simulink model "playback_data"  (R2015a)
settings: Solver=FixedStepDiscrete  SolverMode=SingleTasking  StartTime=44  StopTime=72  FixedStep=sample_time  RelTol=1e-3
undefined symbols (not defined in the file or in its folder): A_kalman_no_position, A_kalman_transverse, A_kalman_vertical, A_lpf_10hz_05d, A_lpf_accelerometer, A_lpf_fourbar_angles, A_lpf_imu, A_lpf_lateral_angle, B1_lpf_10hz_05d, B1_lpf_accelerometer, B1_lpf_fourbar_angles, B1_lpf_imu, B1_lpf_lateral_angle, B2_lpf_10hz_05d, B2_lpf_accelerometer, B2_lpf_fourbar_angles, B2_lpf_imu, B2_lpf_lateral_angle, B_dx_versus_x0, B_kalman_no_position, B_kalman_transverse, B_kalman_vertical, backwards_K_sag_of_t, backwards_P_sag_of_t, boom_mount_angle, C_kalman_no_position, C_kalman_transverse, C_kalman_vertical, com_leg_motor, com_torso, contact_threshold, control_start_time, d_ankle_to_foot, d_vertical_boom_com_offset, d_vertical_com, desired_com_forward_velocity, desired_com_lateral_velocity, desired_initial_leg_roll_left, desired_initial_leg_roll_right, desired_standing_torso_pitch, desired_standing_torso_roll, desired_standing_z, desired_torso_pitch, desired_torso_roll, Discrete, enable_bouncing, fcut_contact, fdesignblkfcn, forward_dx_of_dxstar, forward_x_of_dxstar, g, gcbh, h_boom, HIP_MTR_MAX_CONT_TORQUE, HIP_MTR_MAX_TORQUE, i_leg_motor, i_robot, i_torso, initial_dx_estimate, initial_dx_takeoff_history ... (+82)
libraries: simulink x23, ctrlSharedLib x4, dsparch4 x3, dspfdesign x1
(part 2 of 6)

== system playback_data/Control/Behavior Control/Atrias Swing control ==
  note: Convert to
      | four-bar angles
  note: Position control the
      | individual four bar segments
  X Desired [m m/s m/s^2] : Inport
  Y Desired [m m/s m/s^2] : Inport  Port=2
  Z Desired [m m/s m/s^2] : Inport  Port=3
  Secondary Front Gear [rad rad/s] : Inport  Port=4
  Secondary Back Gear [rad rad/s] : Inport  Port=5
  Right or Left Stance [1 or 0] : Inport  Port=6
  Secondary Leg Roll [rad rad/s] : Inport  Port=7
  Secondary Leg Length [m m/s] : Inport  Port=8
  Secondary Leg Angle [rad rad/s] : Inport  Port=9
  Torso Pitch [rad rad/s] : Inport  Port=10
  Torso Roll [rad rad/s] : Inport  Port=11
  Pelvis to COM Position [m m m] : Inport  Port=12
  Pelvis to COM Velocity [m/s m/s m/s] : Inport  Port=13
  Avoid Hitting Mechanical Limits : MATLAB Function  TreatAsAtomicUnit=on
  Back / Front Velocity Tracking : Scope  NumInputPorts=2
      settings: YMin=-0.75~-5  YMax=3.25~1.5  SaveName=ScopeData36  SampleInput=on
  Back/Front PD : Subsystem
  "Convert COM Position to Joint Angles + Leg Length " : MATLAB Function  TreatAsAtomicUnit=on
  Demux4 : Demux  Outputs=2
  Demux5 : Demux  Outputs=2
  Demux6 : Demux  Outputs=6
  Mux{3..6,8,11..13} (8 alike) : Mux  Inputs=2
  Selector1 : Selector  InputPortWidth=2  Indices=[1]
  Selector2 : Selector  InputPortWidth=2  Indices=[1]
  Selector7 : Selector  InputPortWidth=2  Indices=[2]
  Selector8 : Selector  InputPortWidth=2  Indices=[2]
  Terminator : Terminator
  Two Pole Filter : DiscreteTransferFcn  Numerator=[A_lpf_10hz_05d 0 0]  Denominator=[1 B1_lpf_10hz_05d B2_lpf_10hz_05d]  SampleTime=sample_time
  Virtual Leg to Four Bar : MATLAB Function  TreatAsAtomicUnit=on
  Secondary Back/Front Motor Velocity [rad/s rad/s] : Outport
  Desired Swing Beta [rad rad/s rad/s^2] : Outport  Port=2
  wires:
  Two Pole Filter/1 -> Secondary Back/Front Motor Velocity [rad/s rad/s]/1
  Selector8/1 -> Mux12/2
  Selector7/1 -> Mux12/1
  Selector2/1 -> Mux13/2
  Selector1/1 -> Mux13/1
  Mux13/1 -> Back / Front Velocity Tracking/1
  Mux12/1 -> Back / Front Velocity Tracking/2
  Back/Front PD/1(Commanded Velocity [rad/s] [back front]) -> Selector2/1, Selector8/1, Two Pole Filter/1
  "Convert COM Position to Joint Angles + Leg Length "/3(desired_beta) -> Desired Swing Beta [rad rad/s rad/s^2]/1
  Pelvis to COM Velocity [m/s m/s m/s]/1 -> "Convert COM Position to Joint Angles + Leg Length "/6(dcom_pelvis_body)
  Pelvis to COM Position [m m m]/1 -> "Convert COM Position to Joint Angles + Leg Length "/5(com_pelvis_body)
  Mux5/1 -> Terminator/1
  Virtual Leg to Four Bar/5(dfront) -> Avoid Hitting Mechanical Limits/5(dfront_desired)
  Y Desired [m m/s m/s^2]/1 -> "Convert COM Position to Joint Angles + Leg Length "/2(Y_star)
  Mux8/1 -> Demux6/1
  "Convert COM Position to Joint Angles + Leg Length "/1(desired_leg_length) -> Mux8/1
  X Desired [m m/s m/s^2]/1 -> "Convert COM Position to Joint Angles + Leg Length "/1(X_star)
  Secondary Leg Length [m m/s]/1 -> "Convert COM Position to Joint Angles + Leg Length "/11(leg_length)
  "Convert COM Position to Joint Angles + Leg Length "/2(desired_alpha) -> Mux8/2
  Secondary Leg Angle [rad rad/s]/1 -> "Convert COM Position to Joint Angles + Leg Length "/9(sagittal_angle)
  Secondary Leg Roll [rad rad/s]/1 -> "Convert COM Position to Joint Angles + Leg Length "/10(lateral_angle)  "swing hip angle (lateral)"
  Right or Left Stance [1 or 0]/1 -> "Convert COM Position to Joint Angles + Leg Length "/4(right_left)
  Torso Roll [rad rad/s]/1 -> "Convert COM Position to Joint Angles + Leg Length "/7(roll)
  Torso Pitch [rad rad/s]/1 -> "Convert COM Position to Joint Angles + Leg Length "/8(pitch)
  Virtual Leg to Four Bar/1(back) -> Avoid Hitting Mechanical Limits/1(back_desired)
  Demux4/2 -> Mux11/2
  Demux6/5 -> Virtual Leg to Four Bar/5(dphi)
  Virtual Leg to Four Bar/4(front) -> Avoid Hitting Mechanical Limits/4(front_desired)
  Demux6/6 -> Virtual Leg to Four Bar/6(ddphi)
  Demux6/3 -> Virtual Leg to Four Bar/3(ddl_leg)
  Demux6/2 -> Virtual Leg to Four Bar/2(dl_leg)
  Virtual Leg to Four Bar/3(ddback) -> Avoid Hitting Mechanical Limits/3(ddback_desired)
  Virtual Leg to Four Bar/6(ddfront) -> Avoid Hitting Mechanical Limits/6(ddfront_desired)
  Mux11/1 -> Selector1/1, Selector7/1
  Virtual Leg to Four Bar/2(dback) -> Avoid Hitting Mechanical Limits/2(dback_desired)
  Demux6/4 -> Virtual Leg to Four Bar/4(phi)
  Demux6/1 -> Virtual Leg to Four Bar/1(l_leg)
  Secondary Back Gear [rad rad/s]/1 -> Demux5/1
  Demux5/1 -> Mux6/1
  Z Desired [m m/s m/s^2]/1 -> "Convert COM Position to Joint Angles + Leg Length "/3(Z_star)
  Mux4/1 -> Back/Front PD/2(Desired Velocity [rad/s] [back front])
  Secondary Front Gear [rad rad/s]/1 -> Demux4/1
  Demux5/2 -> Mux11/1
  Avoid Hitting Mechanical Limits/3(dback_cmd) -> Mux4/1
  Mux3/1 -> Back/Front PD/1(Desired Position [rad] [back front])
  Mux6/1 -> Back/Front PD/3(Measured Position [rad] [back front])
  Avoid Hitting Mechanical Limits/6(ddfront_cmd) -> Mux5/2
  Avoid Hitting Mechanical Limits/5(ddback_cmd) -> Mux5/1
  Avoid Hitting Mechanical Limits/2(front_cmd) -> Mux3/2
  Avoid Hitting Mechanical Limits/4(dfront_cmd) -> Mux4/2
  Avoid Hitting Mechanical Limits/1(back_cmd) -> Mux3/1
  Demux4/1 -> Mux6/2

== system playback_data/Control/Behavior Control/Compute Forces1 ==
  XYZ Acceleration : Inport
  Constant5 : Constant  Value=g
  Demux : Demux  Outputs=3
  Gain4 : Gain  Gain=m_total_real
  Mux : Mux  Inputs=3
  Sum8 : Sum  Inputs=|++
  XYZ Force : Outport
  wires:
  Demux/1 -> Mux/1
  Demux/2 -> Mux/2
  Demux/3 -> Sum8/1
  Sum8/1 -> Mux/3
  Mux/1 -> Gain4/1
  Gain4/1 -> XYZ Force/1
  XYZ Acceleration/1 -> Demux/1
  Constant5/1 -> Sum8/2

== system playback_data/Control/Behavior Control/Contact State Machine ==
  Contact Factor [body weight] : Inport
  "[Z dZ] [m m/s]" : Inport  Port=2
  ddZ [m/s^2] : Inport  Port=3
  Detect Fall Nonpositive : simulink/Logic and Bit Operations/Detect Fall Nonpositive  vinit=1  InputProcessing=Inherited  OutDataTypeStr=boolean
  Flight / Exiting Stance : Scope  NumInputPorts=2
      settings: YMin=0.95~0.95  YMax=1.05~1.05  SaveName=ScopeData54  SampleInput=on
  Mux25 : Mux  Inputs=5
  Selector : Selector  InputPortWidth=2  Indices=[2]
  State Machine : State Transition Table  TreatAsAtomicUnit=on
  Terminator8 : Terminator
  Unit Delay5 : UnitDelay  SampleTime=-1
  Unit Delay6 : UnitDelay  SampleTime=sample_time
  Unit Delay7 : UnitDelay  InitialCondition=1  SampleTime=sample_time
  Unit Delay8 : UnitDelay  SampleTime=sample_time
  flight [1/0] : Outport
  Exiting Stance [1/0] : Outport  Port=2
  wires:
  Detect Fall Nonpositive/1 -> Exiting Stance [1/0]/1, Flight / Exiting Stance/2
  Unit Delay7/1 -> flight [1/0]/1, Flight / Exiting Stance/1
  Unit Delay6/1 -> Detect Fall Nonpositive/1
  State Machine/4(" Takeoff") -> Unit Delay6/1, Mux25/4
  Unit Delay8/1 -> Terminator8/1
  Selector/1 -> State Machine/1(z_velocity), Unit Delay5/1
  Contact Factor [body weight]/1 -> State Machine/3(vertical_grf)
  Unit Delay5/1 -> State Machine/2(previous_z_velocity)
  State Machine/5(" Flight") -> Mux25/5, Unit Delay7/1
  Mux25/1 -> Unit Delay8/1
  State Machine/3(" Unloading") -> Mux25/3
  State Machine/2(" LockedContact") -> Mux25/2
  State Machine/1(" TouchDown") -> Mux25/1
  "[Z dZ] [m m/s]"/1 -> Selector/1
  ddZ [m/s^2]/1 -> State Machine/4(vertical_acceleration)

== system playback_data/Control/Behavior Control/Desired Secondary Swing Targets ==
  Primary X,Y,Z : Inport
  Right / Left : Inport  Port=2
  Primary dX,dY,dZ : Inport  Port=3
  Constant1 : Constant  Value=[lateral_target_position_right, 0]
  Constant2 : Constant  Value=[lateral_target_position_left, 0]
  Constant3 : Constant  Value=[z_retract_swing, 0]
  Constant4 : Constant  Value=0
  Constant5 : Constant  Value=0
  Constant6 : Constant  Value=0
  Demux1 : Demux  Outputs=3
  Demux2 : Demux  Outputs=3
  Demux3 : Demux  Outputs=3
  Desired XYZ : Scope  NumInputPorts=4
      settings: YMin=-0.225~-0.15~0.5~-5  YMax=0.25~0.15~0.875~5  SaveName=ScopeData54  SampleInput=on
  Gain : Gain  Gain=-1
  Mux{25,29,32,34..35} (5 alike) : Mux  Inputs=2
  Primary XYZ : Scope  NumInputPorts=3
      settings: YMin=-0.75~-5~-5  YMax=3.25~1.5~5  SaveName=ScopeData55  SampleInput=on
  Selector3 : Selector  InputPortWidth=3  Indices=[1]
  Selector4 : Selector  InputPortWidth=3  Indices=[1]
  Selector5 : Selector  InputPortWidth=3  Indices=[1]
  Sum2 : Sum  Inputs=-+|
  Switch1 : Switch  Criteria=u2 ~= 0
  Terminator : Terminator
  Terminator1 : Terminator
  Desired X : Outport
  Desired Y : Outport  Port=2
  Desired Z : Outport  Port=3
  wires:
  Demux3/3 -> Primary XYZ/3
  Demux3/2 -> Primary XYZ/2
  Demux3/1 -> Primary XYZ/1
  Selector4/1 -> Desired XYZ/2
  Selector5/1 -> Desired XYZ/3
  Selector3/1 -> Desired XYZ/1
  Mux32/1 -> Desired X/1, Selector3/1
  Mux25/1 -> Desired Y/1, Selector4/1
  Mux29/1 -> Desired Z/1, Selector5/1
  Mux35/1 -> Sum2/2
  Constant3/1 -> Sum2/1
  Sum2/1 -> Mux29/1
  Constant2/1 -> Switch1/1
  Constant1/1 -> Switch1/3
  Right / Left/1 -> Switch1/2, Desired XYZ/4
  Switch1/1 -> Mux25/1
  Constant4/1 -> Mux32/2
  Constant5/1 -> Mux25/2
  Constant6/1 -> Mux29/2
  Gain/1 -> Mux32/1
  Primary X,Y,Z/1 -> Demux1/1, Demux3/1
  Primary dX,dY,dZ/1 -> Demux2/1
  Demux2/1 -> Mux34/2
  Demux1/1 -> Mux34/1
  Demux1/2 -> Terminator1/1
  Mux34/1 -> Gain/1
  Demux1/3 -> Mux35/1
  Demux2/3 -> Mux35/2
  Demux2/2 -> Terminator/1

== system playback_data/Control/Behavior Control/Estimate Angular Accelerations2 ==
  Angular Velocities [rad/s] x3 : Inport
  Enabled : Inport  Port=2
  Detect Change : simulink/Logic and Bit Operations/Detect Change  vinit=0  InputProcessing=Inherited  OutDataTypeStr=boolean
  Difference : simulink/Discrete/Difference  ICPrevInput=0.0  InputProcessing=Inherited  OutMin=[]  OutMax=[]  OutDataType=fixdt(1, 16)  OutScaling=2^-10  DoSatur=off
  Gain : Gain  Gain=1/sample_time
  IMU Two Pole Filter1 : DiscreteTransferFcn  Numerator=[A_lpf_imu 0 0]  Denominator=[1 B1_lpf_imu B2_lpf_imu]  SampleTime=sample_time
  Logical Operator5 : Logic  Operator=NOT  AllPortsSameDT=off  OutDataTypeStr=boolean
  Product : Product
  Angular Accelerations [rad/s^2] x3 : Outport
  wires:
  Enabled/1 -> Detect Change/1
  Logical Operator5/1 -> Product/2
  Product/1 -> IMU Two Pole Filter1/1
  Angular Velocities [rad/s] x3/1 -> Difference/1
  Gain/1 -> Product/1
  Difference/1 -> Gain/1
  Detect Change/1 -> Logical Operator5/1
  IMU Two Pole Filter1/1 -> Angular Accelerations [rad/s^2] x3/1

== system playback_data/Control/Behavior Control/Estimate Angular Accelerations3 ==
  Angular Velocities [rad/s] x2 : Inport
  Enabled : Inport  Port=2
  Detect Change : simulink/Logic and Bit Operations/Detect Change  vinit=0  InputProcessing=Inherited  OutDataTypeStr=boolean
  Difference : simulink/Discrete/Difference  ICPrevInput=0.0  InputProcessing=Inherited  OutMin=[]  OutMax=[]  OutDataType=fixdt(1, 16)  OutScaling=2^-10  DoSatur=off
  Gain : Gain  Gain=1/sample_time
  Lateral Angle Two Pole Filter1 : DiscreteTransferFcn  Numerator=[A_lpf_lateral_angle 0 0]  Denominator=[1 B1_lpf_lateral_angle B2_lpf_lateral_angle]  SampleTime=sample_time
  Logical Operator5 : Logic  Operator=NOT  AllPortsSameDT=off  OutDataTypeStr=boolean
  Product : Product
  Angular Accelerations [rad/s^2] x2 : Outport
  wires:
  Detect Change/1 -> Logical Operator5/1
  Difference/1 -> Gain/1
  Gain/1 -> Product/1
  Angular Velocities [rad/s] x2/1 -> Difference/1
  Product/1 -> Lateral Angle Two Pole Filter1/1
  Logical Operator5/1 -> Product/2
  Enabled/1 -> Detect Change/1
  Lateral Angle Two Pole Filter1/1 -> Angular Accelerations [rad/s^2] x2/1

== system playback_data/Control/Behavior Control/Exited Stance ==
  Enable : EnablePort  StatesWhenEnabling=reset
  Constant : Constant
  Takeoff? : Outport  InitialOutput=[0]
  wires:
  Constant/1 -> Takeoff?/1

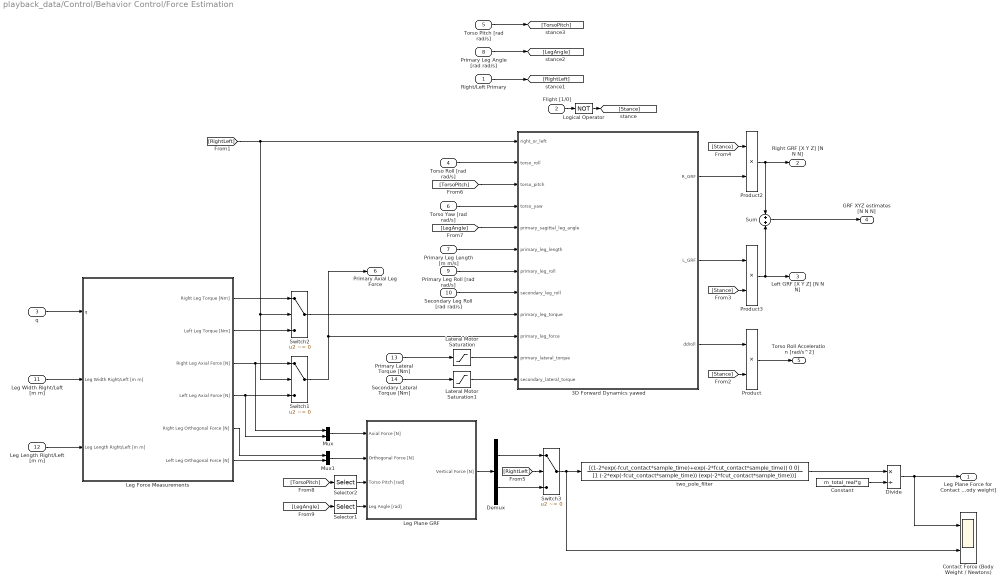
== system playback_data/Control/Behavior Control/Force Estimation ==
  Right/Left Primary : Inport
  Flight [1/0] : Inport  Port=2
  q : Inport  Port=3
  Torso Roll [rad rad/s] : Inport  Port=4
  Torso Pitch [rad rad/s] : Inport  Port=5
  Torso Yaw [rad rad/s] : Inport  Port=6
  Primary Leg Length [m m/s] : Inport  Port=7
  Primary Leg Angle [rad rad/s] : Inport  Port=8
  Primary Leg Roll [rad rad/s] : Inport  Port=9
  Secondary Leg Roll [rad rad/s] : Inport  Port=10
  Leg Width Right/Left [m m] : Inport  Port=11
  Leg Length Right/Left [m m] : Inport  Port=12
  Primary Lateral Torque [Nm] : Inport  Port=13
  Secondary Lateral Torque [Nm] : Inport  Port=14
  3D Forward Dynamics yawed : MATLAB Function  TreatAsAtomicUnit=on
  Constant : Constant  Value=m_total_real*g
  Contact Force (Body Weight / Newtons) : Scope  NumInputPorts=2
      settings: YMin=1~1  YMax=1~1  SaveName=ScopeData49  SampleInput=on
  Demux : Demux  Outputs=2
  Divide : Product  Inputs=*/
  Lateral Motor Saturation : Saturate  UpperLimit=HIP_MTR_MAX_TORQUE  LowerLimit=-HIP_MTR_MAX_TORQUE
      settings: AttributesFormatString=Top: %<UpperLimit>\nBottom: %<LowerLimit>
  Lateral Motor Saturation1 : Saturate  UpperLimit=HIP_MTR_MAX_TORQUE  LowerLimit=-HIP_MTR_MAX_TORQUE
      settings: AttributesFormatString=Top: %<UpperLimit>\nBottom: %<LowerLimit>
  Leg Force Measurements : Subsystem
  Leg Plane GRF : Subsystem
  Logical Operator : Logic  Operator=NOT  AllPortsSameDT=off  OutDataTypeStr=boolean
  Mux : Mux  Inputs=2
  Mux1 : Mux  Inputs=2
  Product : Product
  Product2 : Product
  Product3 : Product
  Selector1 : Selector  InputPortWidth=2  Indices=[1]
  Selector2 : Selector  InputPortWidth=2  Indices=[1]
  Sum : Sum  Inputs=+|+
  Switch1 : Switch  Criteria=u2 ~= 0
  Switch2 : Switch  Criteria=u2 ~= 0
  Switch3 : Switch  Criteria=u2 ~= 0
  two_pole_filter : DiscreteTransferFcn  Numerator=[(1-2*exp(-fcut_contact*sample_time)+exp(-2*fcut_contact*sample_time)) 0 0]  Denominator=[1 (-2*exp(-fcut_contact*sample_time)) (exp(-2*fcut_contact*sample_time))]  SampleTime=sample_time
  Leg Plane Force for Contact Detection [body weight] : Outport
  Right GRF [X Y Z] [N N N] : Outport  Port=2
  Left GRF [X Y Z] [N N N] : Outport  Port=3
  GRF XYZ estimates [N N N] : Outport  Port=4  OutputWhenDisabled=reset  InitialOutput=[0 0 0 0 0 0]
  Torso Roll Acceleration [rad/s^2] : Outport  Port=5  OutputWhenDisabled=reset  InitialOutput=[0 0 0 0 0 0]
  Primary Axial Leg Force : Outport  Port=6
  wires:
  Divide/1 -> Leg Plane Force for Contact Detection [body weight]/1, Contact Force (Body Weight / Newtons)/1
  Leg Width Right/Left [m m]/1 -> Leg Force Measurements/2(Leg Width Right/Left [m m])
  q/1 -> Leg Force Measurements/1(q)
  two_pole_filter/1 -> Divide/1
  Constant/1 -> Divide/2
  [RightLeft] -> 3D Forward Dynamics yawed/1(right_or_left), Switch2/2, Switch1/2
  Leg Length Right/Left [m m]/1 -> Leg Force Measurements/3(Leg Length Right/Left [m m])
  3D Forward Dynamics yawed/1(R_GRF) -> Product2/2
  3D Forward Dynamics yawed/2(L_GRF) -> Product3/1
  3D Forward Dynamics yawed/3(ddroll) -> Product/1
  Leg Force Measurements/3(Right Leg Axial Force [N]) -> Mux/1, Switch1/1
  Leg Force Measurements/4(Left Leg Axial Force [N]) -> Switch1/3, Mux/2
  Switch1/1 -> Primary Axial Leg Force/1, 3D Forward Dynamics yawed/10(primary_leg_force)
  [TorsoPitch] -> 3D Forward Dynamics yawed/3(torso_pitch)
  Torso Roll [rad rad/s]/1 -> 3D Forward Dynamics yawed/2(torso_roll)
  Torso Yaw [rad rad/s]/1 -> 3D Forward Dynamics yawed/4(torso_yaw)
  Primary Leg Length [m m/s]/1 -> 3D Forward Dynamics yawed/6(primary_leg_length)
  [LegAngle] -> 3D Forward Dynamics yawed/5(primary_sagittal_leg_angle)
  Flight [1/0]/1 -> Logical Operator/1
  [Stance] -> Product/2
  Product/1 -> Torso Roll Acceleration [rad/s^2]/1
  Switch3/1 -> two_pole_filter/1, Contact Force (Body Weight / Newtons)/2
  Logical Operator/1 -> [Stance]
  Product3/1 -> Left GRF [X Y Z] [N N N]/1, Sum/2
  Product2/1 -> Right GRF [X Y Z] [N N N]/1, Sum/1
  [Stance] -> Product3/2
  [Stance] -> Product2/1
  Primary Leg Roll [rad rad/s]/1 -> 3D Forward Dynamics yawed/7(primary_leg_roll)
  Secondary Leg Roll [rad rad/s]/1 -> 3D Forward Dynamics yawed/8(secondary_leg_roll)
  Switch2/1 -> 3D Forward Dynamics yawed/9(primary_leg_torque)
  Leg Force Measurements/1(Right Leg Torque [Nm]) -> Switch2/1
  Leg Force Measurements/2(Left Leg Torque [Nm]) -> Switch2/3
  Sum/1 -> GRF XYZ estimates [N N N]/1
  Mux1/1 -> Leg Plane GRF/2(Orthogonal Force [N])
  Mux/1 -> Leg Plane GRF/1(Axial Force [N])
  Leg Force Measurements/5(Right Leg Orthogonal Force [N]) -> Mux1/1
  Leg Force Measurements/6(Left Leg Orthogonal Force [N]) -> Mux1/2
  Right/Left Primary/1 -> [RightLeft]
  [RightLeft] -> Switch3/2
  Leg Plane GRF/1(Vertical Force [N]) -> Demux/1
  Demux/1 -> Switch3/1
  Demux/2 -> Switch3/3
  Primary Leg Angle [rad rad/s]/1 -> [LegAngle]
  Torso Pitch [rad rad/s]/1 -> [TorsoPitch]
  [LegAngle] -> Selector1/1
  Selector1/1 -> Leg Plane GRF/4(Leg Angle [rad])
  [TorsoPitch] -> Selector2/1
  Selector2/1 -> Leg Plane GRF/3(Torso Pitch [rad])
  Primary Lateral Torque [Nm]/1 -> Lateral Motor Saturation/1
  Secondary Lateral Torque [Nm]/1 -> Lateral Motor Saturation1/1
  Lateral Motor Saturation/1 -> 3D Forward Dynamics yawed/11(primary_lateral_torque)
  Lateral Motor Saturation1/1 -> 3D Forward Dynamics yawed/12(secondary_lateral_torque)

== system playback_data/Control/Behavior Control/L Leg Calculator ==
  Front [rad rad/s] : Inport
  Back [rad rad/s] : Inport  Port=2
  Constant : Constant  Value=d_ankle_to_foot-0.01
  Demux1 : Demux  Outputs=2
  Gain1 : Gain  Gain=2*l_seg
  Gain2 : Gain  Gain=l_seg
  Gain3 : Gain  Gain=-1
  Gain4 : Gain  Gain=0.5
  Gain5 : Gain  Gain=0.5
  Gain6 : Gain  Gain=2
  Mux1 : Mux  Inputs=2
  Product : Product  RndMeth=Zero
  Sum : Sum  Inputs=++|
  Sum4 : Sum  Inputs=+|+
  Sum5 : Sum  Inputs=+|-
  Trigonometric Function : Trigonometry  Operator=cos
  Trigonometric Function1 : Trigonometry
  "Leg Length [m m/s] " : Outport
  Leg Angle [rad rad/s] : Outport  Port=2
  Leg Splay [rad rad/s] : Outport  Port=3
  w [m] : Outport  Port=4
  wires:
  Sum/1 -> Mux1/1
  Sum4/1 -> Gain5/1
  Mux1/1 -> "Leg Length [m m/s] "/1
  Sum5/1 -> Demux1/1, Leg Splay [rad rad/s]/1
  Gain2/1 -> Gain6/1, Product/1
  Demux1/1 -> Gain4/1
  Gain3/1 -> Product/2
  Demux1/2 -> Gain3/1
  Back [rad rad/s]/1 -> Sum5/1, Sum4/1
  Front [rad rad/s]/1 -> Sum4/2, Sum5/2
  Product/1 -> Mux1/2
  Trigonometric Function1/1 -> Gain2/1
  Gain1/1 -> Sum/2
  Trigonometric Function/1 -> Gain1/1
  Gain4/1 -> Trigonometric Function/1, Trigonometric Function1/1
  Gain6/1 -> w [m]/1
  Gain5/1 -> Leg Angle [rad rad/s]/1

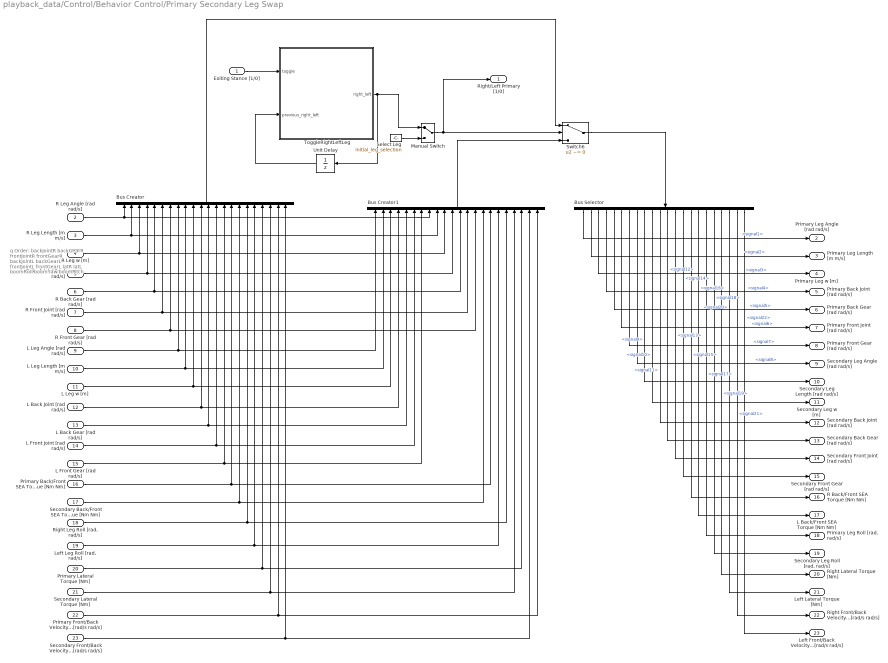
== system playback_data/Control/Behavior Control/Primary Secondary Leg Swap ==
  note: q Order:
      |
      | backJointR
      | backGearR
      | frontJointR
      | frontGearR
      |
      | backJointL
      | backGearL
      | frontJointL
      | frontGearL
      |
      | latR
      | latL
      |
      | boomRoll
      | boomYaw
      | boomPitch
  Exiting Stance [1/0] : Inport
  R Leg Angle [rad rad/s] : Inport  Port=2
  R Leg Length [m m/s] : Inport  Port=3
  R Leg w [m] : Inport  Port=4
  R Back Joint [rad rad/s] : Inport  Port=5
  R Back Gear [rad rad/s] : Inport  Port=6
  R Front Joint [rad rad/s] : Inport  Port=7
  R Front Gear [rad rad/s] : Inport  Port=8
  L Leg Angle [rad rad/s] : Inport  Port=9
  L Leg Length [m m/s] : Inport  Port=10
  L Leg w [m] : Inport  Port=11
  L Back Joint [rad rad/s] : Inport  Port=12
  L Back Gear [rad rad/s] : Inport  Port=13
  L Front Joint [rad rad/s] : Inport  Port=14
  L Front Gear [rad rad/s] : Inport  Port=15
  Primary Back/Front SEA Torque [Nm Nm] : Inport  Port=16
  Secondary Back/Front SEA Torque [Nm Nm] : Inport  Port=17
  "Right Leg Roll [rad, rad/s]" : Inport  Port=18
  "Left Leg Roll [rad, rad/s]" : Inport  Port=19
  Primary Lateral Torque [Nm] : Inport  Port=20
  Secondary Lateral Torque [Nm] : Inport  Port=21
  Primary Front/Back Velocity [rad/s rad/s] : Inport  Port=22
  Secondary Front/Back Velocity [rad/s rad/s] : Inport  Port=23
  Bus Creator : BusCreator  Inputs=22
  Bus Creator1 : BusCreator  Inputs=22
  Bus Selector : BusSelector  OutputSignals=signal1,signal2,signal3,signal4,signal5,signal6,signal7,signal8,signal9,signal10,signal11,signal12,signal13,signal14,signal15,signal16,signal17,signal18,signal19,signal20,signal21,signal22
  Manual Switch : ManualSwitch
  Select Leg : Constant  Value=initial_leg_selection  OutDataTypeStr=boolean
  Switch6 : Switch  Criteria=u2 ~= 0  OutDataTypeStr=Inherit: Inherit via back propagation  ZeroCross=off
  ToggleRightLeftLeg : MATLAB Function  TreatAsAtomicUnit=on
      settings: MinAlgLoopOccurrences=on
  Unit Delay : UnitDelay  InitialCondition=initial_leg_selection  SampleTime=sample_time
  Right/Left Primary [1/0] : Outport
  Primary Leg Angle [rad rad/s] : Outport  Port=2
  Primary Leg Length [m m/s] : Outport  Port=3
  Primary Leg w [m] : Outport  Port=4
  Primary Back Joint [rad rad/s] : Outport  Port=5
  Primary Back Gear [rad rad/s] : Outport  Port=6
  Primary Front Joint [rad rad/s] : Outport  Port=7
  Primary Front Gear [rad rad/s] : Outport  Port=8
  Secondary Leg Angle [rad rad/s] : Outport  Port=9
  Secondary Leg Length [rad rad/s] : Outport  Port=10
  Secondary Leg w [m] : Outport  Port=11
  Secondary Back Joint [rad rad/s] : Outport  Port=12
  Secondary Back Gear [rad rad/s] : Outport  Port=13
  Secondary Front Joint [rad rad/s] : Outport  Port=14
  Secondary Front Gear [rad rad/s] : Outport  Port=15
  R Back/Front SEA Torque [Nm Nm] : Outport  Port=16
  L Back/Front SEA Torque [Nm Nm] : Outport  Port=17
  "Primary Leg Roll [rad, rad/s]" : Outport  Port=18
  "Secondary Leg Roll [rad, rad/s]" : Outport  Port=19
  Right Lateral Torque [Nm] : Outport  Port=20
  Left Lateral Torque [Nm] : Outport  Port=21
  Right Front/Back Velocity [rad/s rad/s] : Outport  Port=22
  Left Front/Back Velocity [rad/s rad/s] : Outport  Port=23
  wires:
  Unit Delay/1 -> ToggleRightLeftLeg/2(previous_right_left)
  Exiting Stance [1/0]/1 -> ToggleRightLeftLeg/1(toggle)
  ToggleRightLeftLeg/1(right_left) -> Unit Delay/1, Manual Switch/1
  Manual Switch/1 -> Right/Left Primary [1/0]/1, Switch6/2
  Select Leg/1 -> Manual Switch/2
  R Leg Angle [rad rad/s]/1 -> Bus Creator1/8, Bus Creator/1
  Bus Creator/1 -> Switch6/1
  Bus Creator1/1 -> Switch6/3
  Switch6/1 -> Bus Selector/1
  R Leg Length [m m/s]/1 -> Bus Creator1/9, Bus Creator/2
  R Leg w [m]/1 -> Bus Creator1/10, Bus Creator/3
  R Back Joint [rad rad/s]/1 -> Bus Creator1/11, Bus Creator/4
  R Front Joint [rad rad/s]/1 -> Bus Creator1/13, Bus Creator/6
  R Front Gear [rad rad/s]/1 -> Bus Creator1/14, Bus Creator/7
  L Leg Angle [rad rad/s]/1 -> Bus Creator/8, Bus Creator1/1
  L Leg Length [m m/s]/1 -> Bus Creator1/2, Bus Creator/9
  L Leg w [m]/1 -> Bus Creator1/3, Bus Creator/10
  L Back Joint [rad rad/s]/1 -> Bus Creator1/4, Bus Creator/11
  L Back Gear [rad rad/s]/1 -> Bus Creator1/5, Bus Creator/12
  L Front Joint [rad rad/s]/1 -> Bus Creator1/6, Bus Creator/13
  L Front Gear [rad rad/s]/1 -> Bus Creator1/7, Bus Creator/14
  Primary Back/Front SEA Torque [Nm Nm]/1 -> Bus Creator1/16, Bus Creator/15
  Secondary Back/Front SEA Torque [Nm Nm]/1 -> Bus Creator1/15, Bus Creator/16
  "Right Leg Roll [rad, rad/s]"/1 -> Bus Creator1/18, Bus Creator/17
  "Left Leg Roll [rad, rad/s]"/1 -> Bus Creator1/17, Bus Creator/18
  Primary Lateral Torque [Nm]/1 -> Bus Creator1/20, Bus Creator/19
  Secondary Lateral Torque [Nm]/1 -> Bus Creator1/19, Bus Creator/20
  R Back Gear [rad rad/s]/1 -> Bus Creator1/12, Bus Creator/5
  Bus Selector/1 -> Primary Leg Angle [rad rad/s]/1  "<signal1>"
  Bus Selector/2 -> Primary Leg Length [m m/s]/1  "<signal2>"
  Bus Selector/3 -> Primary Leg w [m]/1  "<signal3>"
  Bus Selector/4 -> Primary Back Joint [rad rad/s]/1  "<signal4>"
  Bus Selector/5 -> Primary Back Gear [rad rad/s]/1  "<signal5>"
  Bus Selector/6 -> Primary Front Joint [rad rad/s]/1  "<signal6>"
  Bus Selector/7 -> Primary Front Gear [rad rad/s]/1  "<signal7>"
  Bus Selector/8 -> Secondary Leg Angle [rad rad/s]/1  "<signal8>"
  Bus Selector/9 -> Secondary Leg Length [rad rad/s]/1  "<signal9>"
  Bus Selector/10 -> Secondary Leg w [m]/1  "<signal10>"
  Bus Selector/11 -> Secondary Back Joint [rad rad/s]/1  "<signal11>"
  Bus Selector/12 -> Secondary Back Gear [rad rad/s]/1  "<signal12>"
  Bus Selector/13 -> Secondary Front Joint [rad rad/s]/1  "<signal13>"
  Bus Selector/14 -> Secondary Front Gear [rad rad/s]/1  "<signal14>"
  Bus Selector/15 -> R Back/Front SEA Torque [Nm Nm]/1  "<signal15>"
  Bus Selector/16 -> L Back/Front SEA Torque [Nm Nm]/1  "<signal16>"
  Bus Selector/17 -> "Primary Leg Roll [rad, rad/s]"/1  "<signal17>"
  Bus Selector/18 -> "Secondary Leg Roll [rad, rad/s]"/1  "<signal18>"
  Bus Selector/19 -> Right Lateral Torque [Nm]/1  "<signal19>"
  Bus Selector/20 -> Left Lateral Torque [Nm]/1  "<signal20>"
  Primary Front/Back Velocity [rad/s rad/s]/1 -> Bus Creator1/22, Bus Creator/21
  Secondary Front/Back Velocity [rad/s rad/s]/1 -> Bus Creator1/21, Bus Creator/22
  Bus Selector/21 -> Right Front/Back Velocity [rad/s rad/s]/1  "<signal21>"
  Bus Selector/22 -> Left Front/Back Velocity [rad/s rad/s]/1  "<signal22>"

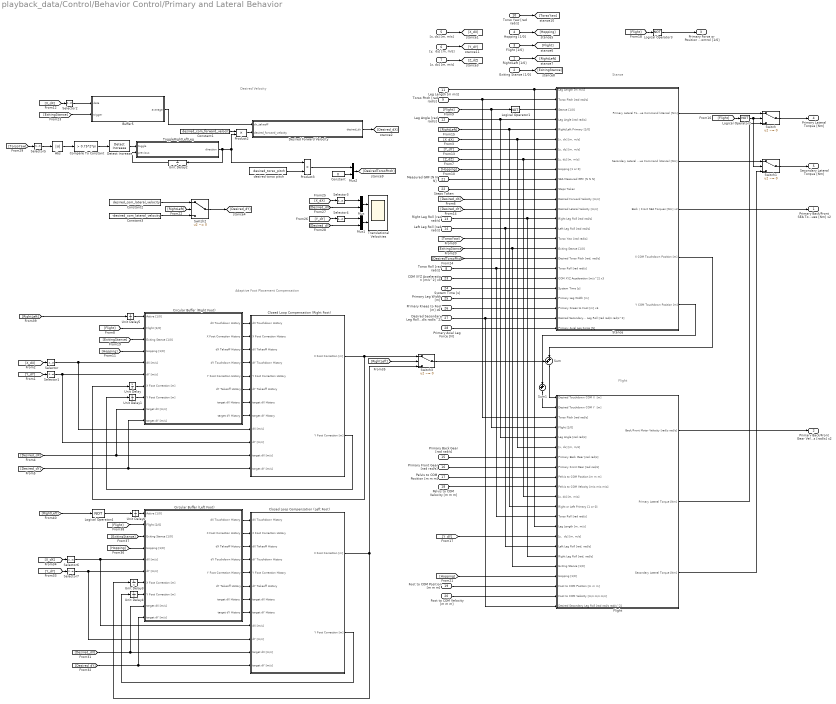
== system playback_data/Control/Behavior Control/Primary and Lateral Behavior ==
  note: Stance
  note: Flight
  note: Adaptive Foot Placement Compensation
  note: Desired Velocity
  Right/Left [1/0] : Inport
  Exiting Stance [1/0] : Inport  Port=2
  Flight [1/0] : Inport  Port=3
  Hopping [1/0] : Inport  Port=4
  "[x, dx] [m, m/s]" : Inport  Port=5
  "[y,  dy] [m, m/s]" : Inport  Port=6
  "[z, dz] [m, m/s]" : Inport  Port=7
  Torso Roll [rad rad/s] : Inport  Port=8
  Torso Pitch [rad rad/s] : Inport  Port=9
  Torso Yaw [rad rad/s] : Inport  Port=10
  Leg Length [m m/s] : Inport  Port=11
  Leg Angle [rad rad/s] : Inport  Port=12
  Right Leg Roll [rad rad/s] : Inport  Port=13
  Left Leg Roll [rad rad/s] : Inport  Port=14
  Primary Back Gear [rad rad/s] : Inport  Port=15
  Primary Front Gear [rad rad/s] : Inport  Port=16
  Pelvis to COM Position [m m m] : Inport  Port=17
  Pelvis to COM Velocity [m m m] : Inport  Port=18
  Foot to COM Position [m m m] : Inport  Port=19
  Foot to COM Velocity [m m m] : Inport  Port=20
  Measured GRF [N N N] : Inport  Port=21
  Steps Taken : Inport  Port=22
  COM XYZ Acceleration [m/s^2] x3 : Inport  Port=23
  System Time [s] : Inport  Port=24
  Primary Leg Width [m] : Inport  Port=25
  Primary Knees to Foot [m] x6 : Inport  Port=26
  Desired Secondary Leg Roll [rad rad/s rad/s^2] : Inport  Port=27
  Primary Axial Leg Force [N] : Inport  Port=28
  Abs : Abs
  Buffer5 : MATLAB Function  TreatAsAtomicUnit=on  SystemSampleTime=sample_time
  Circular Buffer (Left Foot) : Subsystem
  Circular Buffer (Right Foot) : Subsystem
  Closed Loop Compensation (Left Foot) : Subsystem
  Closed Loop Compensation (Right Foot) : Subsystem
  Compare To Constant : simulink/Logic and Bit Operations/Compare To Constant  relop=>  const=0.75*2*pi  OutDataTypeStr=boolean
  Constant : Constant  Value=0
  Constant1 : Constant  Value=desired_com_forward_velocity
  Constant2 : Constant  Value=desired_com_lateral_velocity
  Constant3 : Constant  Value=-desired_com_lateral_velocity
  Desired Forward Velocity : MATLAB Function  TreatAsAtomicUnit=on
  Detect Increase : simulink/Logic and Bit Operations/Detect Increase  vinit=0.0  InputProcessing=Inherited  OutDataTypeStr=boolean
  Flight : Subsystem
  Logical Operator{1..4} (4 alike) : Logic  Operator=NOT  AllPortsSameDT=off  OutDataTypeStr=boolean
  Mux : Mux  Inputs=2
  Mux1 : Mux  Inputs=2
  Mux2 : Mux  Inputs=2
  Product2 : Product
  Product3 : Product
  Selector{,1..4,6..7} (7 alike) : Selector  InputPortWidth=2  Indices=[2]
  Selector5 : Selector  InputPortWidth=2  Indices=[1]
  Stance : Subsystem
  Sum : Sum  Inputs=++|
  Sum1 : Sum  Inputs=++|
  Switch{,1..3} (4 alike) : Switch  Criteria=u2 ~= 0
  ToggleRightLeftLeg : MATLAB Function  TreatAsAtomicUnit=on
      settings: MinAlgLoopOccurrences=on
  Translational Velocities : Scope  NumInputPorts=2
      settings: YMin=-1000~-5  YMax=1000~5  SaveName=ScopeData2  SampleInput=on
  Unit Delay{,1,3..6} (6 alike) : UnitDelay  SampleTime=-1
  Unit Delay2 : UnitDelay  InitialCondition=1  SampleTime=sample_time
  desired torso pitch : Constant  Value=desired_torso_pitch
  Primary Back/Front SEA Torques [Nm] x2 : Outport
  Primary Back/Front Gear Velocities [rad/s] x2 : Outport  Port=2
  Primary Force or Position Control [1/0] : Outport  Port=3  OutDataTypeStr=boolean
  Primary Lateral Torque [Nm] : Outport  Port=4
  Secondary Lateral Torque [Nm] : Outport  Port=5
  wires:
  Unit Delay6/1 -> Circular Buffer (Left Foot)/1(Active [1/0])
  Unit Delay5/1 -> Circular Buffer (Right Foot)/1(Active [1/0])
  [RightLeft] -> Logical Operator4/1
  Logical Operator4/1 -> Unit Delay6/1
  [RightLeft] -> Unit Delay5/1
  [Hopping] -> Circular Buffer (Left Foot)/4(Hopping [1/0])
  [ExitingStance] -> Circular Buffer (Left Foot)/3(Exiting Stance [1/0])
  [Flight] -> Circular Buffer (Left Foot)/2(Flight [1/0])
  [RightLeft] -> Switch3/2
  Switch3/1 -> Sum/1
  Selector7/1 -> Closed Loop Compensation (Left Foot)/10(dY [m/s]), Circular Buffer (Left Foot)/6(dY [m/s])
  Selector6/1 -> Closed Loop Compensation (Left Foot)/9(dX [m/s]), Circular Buffer (Left Foot)/5(dX [m/s])
  [X_dX] -> Selector6/1
  [Y_dY] -> Selector7/1
  [Desired_dX] -> Closed Loop Compensation (Left Foot)/11(target dX [m/s]), Circular Buffer (Left Foot)/9(target dX [m/s])
  [Desired_dY] -> Circular Buffer (Left Foot)/10(target dY [m/s]), Closed Loop Compensation (Left Foot)/12("target dY [m/s] ")
  Closed Loop Compensation (Left Foot)/2(Y Foot Correction [m]) -> Unit Delay4/1
  Closed Loop Compensation (Left Foot)/1(X Foot Correction [m]) -> Switch3/3, Unit Delay3/1
  Unit Delay4/1 -> Circular Buffer (Left Foot)/8(Y Foot Correction [m])
  Unit Delay3/1 -> Circular Buffer (Left Foot)/7(X Foot Correction [m])
  Circular Buffer (Left Foot)/3(dX Takeoff History) -> Closed Loop Compensation (Left Foot)/3(dX Takeoff History)
  Circular Buffer (Left Foot)/2(X Foot Correction History) -> Closed Loop Compensation (Left Foot)/2(X Foot Correction History)
  Circular Buffer (Left Foot)/1("dX Touchdown History ") -> Closed Loop Compensation (Left Foot)/1(dX Touchdown History)
  Circular Buffer (Left Foot)/4("dY Touchdown History ") -> Closed Loop Compensation (Left Foot)/4(dY Touchdown History)
  Circular Buffer (Left Foot)/5(Y Foot Correction History) -> Closed Loop Compensation (Left Foot)/5(Y Foot Correction History)
  Circular Buffer (Left Foot)/6(dY Takeoff History) -> Closed Loop Compensation (Left Foot)/6(dY Takeoff History)
  Circular Buffer (Left Foot)/8(target dY History) -> Closed Loop Compensation (Left Foot)/8(target dY History)
  Circular Buffer (Left Foot)/7(target dX History) -> Closed Loop Compensation (Left Foot)/7(target dX History)
  [ExitingStance] -> Buffer5/2(trigger)
  Selector2/1 -> Buffer5/1(data)
  Abs/1 -> Compare To Constant/1
  Constant/1 -> Mux2/2
  Mux2/1 -> [DesiredTorsoPitch]
  [TorsoYaw] -> Selector5/1
  Detect Increase/1 -> ToggleRightLeftLeg/1(toggle)
  Compare To Constant/1 -> Detect Increase/1
  Selector5/1 -> Abs/1
  Torso Yaw [rad rad/s]/1 -> [TorsoYaw]
  Primary Axial Leg Force [N]/1 -> Stance/25(Primary Axial Leg Force [N])
  Desired Secondary Leg Roll [rad rad/s rad/s^2]/1 -> Flight/22(Desired Secondary Leg Roll [rad rad/s rad/s^2]), Stance/24(Desired Secondary Leg Roll [rad rad/s rad/s^2])
  Leg Length [m m/s]/1 -> Stance/1(Leg Length [m m/s]), Flight/14("Leg Length [m, m/s]")
  Torso Pitch [rad rad/s]/1 -> Stance/2(Torso Pitch [rad rad/s]), Flight/3(Torso Pitch [rad rad/s])
  [Hopping] -> Stance/9(Hopping [1 or 0])
  [X_dX] -> Stance/6("[x, dx] [m, m/s]"), Flight/6("[x, dx] [m, m/s]")
  [RightLeft] -> Stance/5(Right/Left Primary [1/0]), Flight/12(Right or Left Primary [1 or 0])
  Primary Back Gear [rad rad/s]/1 -> Flight/7(Primary Back Gear [rad rad/s])
  Primary Front Gear [rad rad/s]/1 -> Flight/8(Primary Front Gear [rad rad/s])
  Leg Angle [rad rad/s]/1 -> Stance/4(Leg Angle [rad rad/s]), Flight/5(Leg Angle [rad rad/s])
  Flight/1(Back/Front Motor Velocity [rad/s rad/s]) -> Primary Back/Front Gear Velocities [rad/s] x2/1
  Logical Operator1/1 -> Stance/3(Stance [1/0])
  [Flight] -> Circular Buffer (Right Foot)/2(Flight [1/0])
  Pelvis to COM Position [m m m]/1 -> Flight/9(Pelvis to COM Position [m m m])
  [Z_dZ] -> Stance/8("[z, dz] [m, m/s]"), Flight/11("[z, dz] [m, m/s]")
  Pelvis to COM Velocity [m m m]/1 -> Flight/10(Pelvis to COM Velocity [m/s m/s m/s])
  Torso Roll [rad rad/s]/1 -> Stance/19(Torso Roll [rad rad/s]), Flight/13(Torso Roll [rad rad/s])
  Measured GRF [N N N]/1 -> Stance/10(SEA Measured GRF [N N N])
  Steps Taken/1 -> Stance/11(Steps Taken)
  [Y_dY] -> Flight/15("[y,  dy] [m, m/s]")
  Circular Buffer (Right Foot)/1("dX Touchdown History ") -> Closed Loop Compensation (Right Foot)/1(dX Touchdown History)
  Circular Buffer (Right Foot)/2(X Foot Correction History) -> Closed Loop Compensation (Right Foot)/2(X Foot Correction History)
  Circular Buffer (Right Foot)/3(dX Takeoff History) -> Closed Loop Compensation (Right Foot)/3(dX Takeoff History)
  Circular Buffer (Right Foot)/4("dY Touchdown History ") -> Closed Loop Compensation (Right Foot)/4(dY Touchdown History)
  Circular Buffer (Right Foot)/5(Y Foot Correction History) -> Closed Loop Compensation (Right Foot)/5(Y Foot Correction History)
  Circular Buffer (Right Foot)/6(dY Takeoff History) -> Closed Loop Compensation (Right Foot)/6(dY Takeoff History)
  Circular Buffer (Right Foot)/8(target dY History) -> Closed Loop Compensation (Right Foot)/8(target dY History)
  Circular Buffer (Right Foot)/7(target dX History) -> Closed Loop Compensation (Right Foot)/7(target dX History)
  [Desired_dX] -> Closed Loop Compensation (Right Foot)/11(target dX [m/s]), Circular Buffer (Right Foot)/9(target dX [m/s])
  [Desired_dY] -> Closed Loop Compensation (Right Foot)/12("target dY [m/s] "), Circular Buffer (Right Foot)/10(target dY [m/s])
  Stance/4(X COM Touchdown Position [m]) -> Sum/2
  Sum/1 -> Flight/1(Desired Touchdown COM X  [m])
  Closed Loop Compensation (Right Foot)/1(X Foot Correction [m]) -> Switch3/1, Unit Delay/1
  Selector1/1 -> Closed Loop Compensation (Right Foot)/10(dY [m/s]), Circular Buffer (Right Foot)/6(dY [m/s])
  Selector/1 -> Closed Loop Compensation (Right Foot)/9(dX [m/s]), Circular Buffer (Right Foot)/5(dX [m/s])
  Unit Delay1/1 -> Circular Buffer (Right Foot)/8(Y Foot Correction [m])
  Unit Delay/1 -> Circular Buffer (Right Foot)/7(X Foot Correction [m])
  Closed Loop Compensation (Right Foot)/2(Y Foot Correction [m]) -> Unit Delay1/1
  "[x, dx] [m, m/s]"/1 -> [X_dX]
  "[z, dz] [m, m/s]"/1 -> [Z_dZ]
  "[y,  dy] [m, m/s]"/1 -> [Y_dY]
  [X_dX] -> Selector/1
  [Y_dY] -> Selector1/1
  [Desired_dX] -> Stance/12(Desired Forward Velocity [m/s])
  Flight [1/0]/1 -> [Flight]
  [Flight] -> Logical Operator1/1, Flight/4(Flight [1/0])
  Hopping [1/0]/1 -> [Hopping]
  Stance/5(Y COM Touchdown Position [m]) -> Sum1/2
  Sum1/1 -> Flight/2(Desired Touchdown COM Y  [m])
  Right Leg Roll [rad rad/s]/1 -> Stance/14(Right Leg Roll [rad rad/s]), Flight/17("Right Leg Roll [rad, rad/s]")
  Left Leg Roll [rad rad/s]/1 -> Flight/16("Left Leg Roll [rad, rad/s]"), Stance/15(Left Leg Roll [rad rad/s])
  [Y_dY] -> Stance/7("[y, dy] [m, m/s]")
  [Desired_dY] -> Stance/13(Desired Lateral Velocity [m/s])
  Right/Left [1/0]/1 -> [RightLeft]
  Logical Operator2/1 -> Switch1/2, Switch/2
  Flight/2(Primary Lateral Torque [Nm]) -> Switch/3
  Flight/3(Secondary Lateral Torque [Nm]) -> Switch1/3
  [Flight] -> Logical Operator2/1
  Switch/1 -> Primary Lateral Torque [Nm]/1
  Switch1/1 -> Secondary Lateral Torque [Nm]/1
  [Flight] -> Logical Operator3/1
  Logical Operator3/1 -> Primary Force or Position Control [1/0]/1
  [TorsoYaw] -> Stance/16(Torso Yaw [rad rad/s])
  [Hopping] -> Circular Buffer (Right Foot)/4(Hopping [1/0])
  [ExitingStance] -> Circular Buffer (Right Foot)/3(Exiting Stance [1/0])
  Exiting Stance [1/0]/1 -> [ExitingStance]
  [ExitingStance] -> Flight/18(Exiting Stance [1/0]), Stance/17(Exiting Stance [1/0])
  [Hopping] -> Flight/19(Hopping [1/0])
  [X_dX] -> Selector2/1
  Switch2/1 -> [Desired_dY]
  Buffer5/1(average) -> Desired Forward Velocity/1(dx_takeoff)
  [RightLeft] -> Switch2/2
  Constant2/1 -> Switch2/1
  Constant3/1 -> Switch2/3
  Desired Forward Velocity/1(desired_dx) -> [Desired_dX]
  Product2/1 -> Desired Forward Velocity/2(desired_forward_velocity)
  ToggleRightLeftLeg/1(direction) -> Product2/2, Product3/1, Unit Delay2/1
  Unit Delay2/1 -> ToggleRightLeftLeg/2(previous)
  Constant1/1 -> Product2/1
  desired torso pitch/1 -> Product3/2
  Product3/1 -> Mux2/1
  [DesiredTorsoPitch] -> Stance/18("Desired Torso Pitch [rad, rad/s]")
  Foot to COM Position [m m m]/1 -> Flight/20(Foot to COM Position [m m m])
  Foot to COM Velocity [m m m]/1 -> Flight/21(Foot to COM Velocity [m/s m/s m/s])
  [X_dX] -> Selector3/1
  Selector3/1 -> Mux/1
  [Y_dY] -> Selector4/1
  Selector4/1 -> Mux1/1
  Mux/1 -> Translational Velocities/1
  Mux1/1 -> Translational Velocities/2
  [Desired_dY] -> Mux1/2
  [Desired_dX] -> Mux/2
  COM XYZ Acceleration [m/s^2] x3/1 -> Stance/20(COM XYZ Acceleration [m/s^2] x3)
  System Time [s]/1 -> Stance/21(System Time [s])
  Primary Leg Width [m]/1 -> Stance/22(Primary Leg Width [m])
  Stance/2(Secondary Lateral Torque Command (stance) [Nm]) -> Switch1/1
  Stance/3(Back / Front SEA Torques [Nm] x2) -> Primary Back/Front SEA Torques [Nm] x2/1
  Stance/1(Primary Lateral Torque Command (stance) [Nm]) -> Switch/1
  Primary Knees to Foot [m] x6/1 -> Stance/23(Primary Knees to Foot [m] x6)

== system playback_data/Control/Behavior Control/R Leg Calculator ==
  Front [rad rad/s] : Inport
  Back [rad rad/s] : Inport  Port=2
  Constant : Constant  Value=d_ankle_to_foot-0.01
  Demux1 : Demux  Outputs=2
  Gain1 : Gain  Gain=2*l_seg
  Gain2 : Gain  Gain=l_seg
  Gain3 : Gain  Gain=-1
  Gain4 : Gain  Gain=0.5
  Gain5 : Gain  Gain=0.5
  Gain6 : Gain  Gain=2
  Mux1 : Mux  Inputs=2
  Product : Product  RndMeth=Zero
  Sum : Sum  Inputs=++|
  Sum4 : Sum  Inputs=+|+
  Sum5 : Sum  Inputs=+|-
  Trigonometric Function : Trigonometry  Operator=cos
  Trigonometric Function1 : Trigonometry
  "Leg Length [m m/s] " : Outport
  Leg Angle [rad rad/s] : Outport  Port=2
  Leg Splay [rad rad/s] : Outport  Port=3
  w [m] : Outport  Port=4
  wires:
  Sum/1 -> Mux1/1
  Gain6/1 -> w [m]/1
  Gain4/1 -> Trigonometric Function1/1, Trigonometric Function/1
  Trigonometric Function/1 -> Gain1/1
  Gain1/1 -> Sum/2
  Trigonometric Function1/1 -> Gain2/1
  Product/1 -> Mux1/2
  Front [rad rad/s]/1 -> Sum5/2, Sum4/2
  Back [rad rad/s]/1 -> Sum4/1, Sum5/1
  Demux1/2 -> Gain3/1
  Gain3/1 -> Product/2
  Demux1/1 -> Gain4/1
  Gain2/1 -> Product/1, Gain6/1
  Sum5/1 -> Leg Splay [rad rad/s]/1, Demux1/1
  Mux1/1 -> "Leg Length [m m/s] "/1
  Sum4/1 -> Gain5/1
  Gain5/1 -> Leg Angle [rad rad/s]/1
